simulink model "SimulinkMorphEUS"  (R2025a)
settings: Solver=VariableStepAuto  StartTime=0.0  StopTime=Tfinal  RelTol=1e-3
values from neighbouring files (symbols this model uses):
  Ixx = 0.246    [SetDroneControl(5).m]    (also in SetDroneControl.m)
  Iyy = 0.336    [SetDroneControl(5).m]    (also in SetDroneControl.m)
  Izz = 0.234    [SetDroneControl(5).m]    (also in SetDroneControl.m)
  lx = 0.2125    [SetDroneControl(5).m]    (also in SetDroneControl.m)
  ly = 0.2125    [SetDroneControl(5).m]    (also in SetDroneControl.m)
  Mass = 3    [SetDroneControl(5).m]    (also in SetDroneControl.m = 5)
libraries: slpidlib x12, matrix_library x8, robotcorelib x4, aerolibobsolete x1, uavutilslib x1
(part 1 of 2)
settings Model: Creator=Nguyen_Duc  LastModifiedBy=Nguyen_Duc

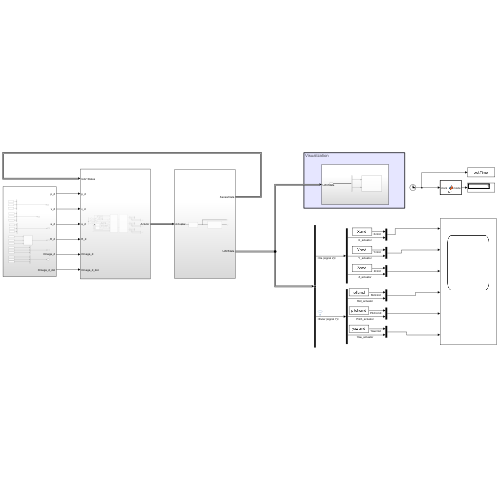
[thumbnail: Simulink's stored preview of the top-level diagram]
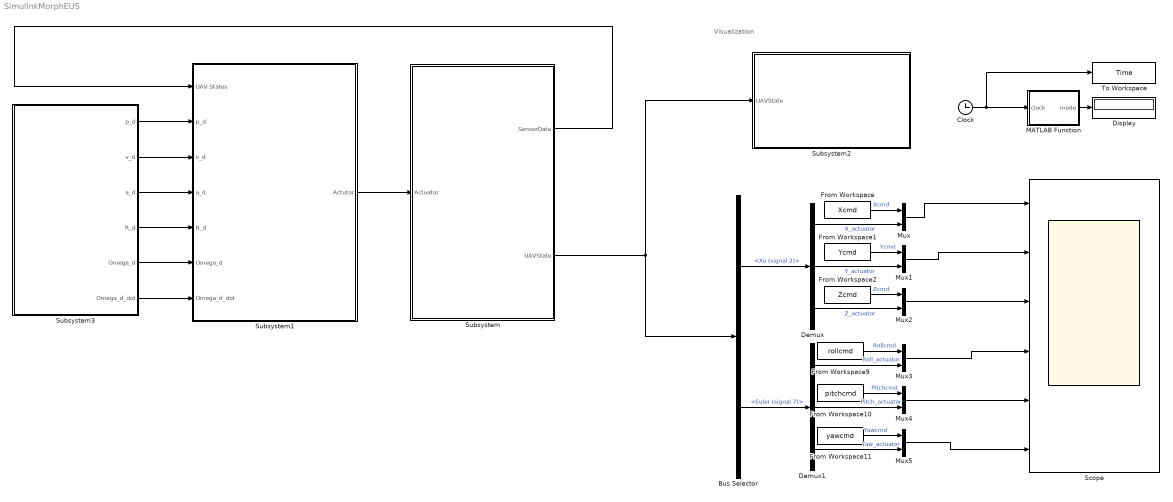
== system SimulinkMorphEUS ==
  note: Visualization
  Bus Selector : BusSelector  OutputSignals=Xe (signal 2),Euler (signal 7)
  Clock : Clock
  Demux : Demux  Outputs=3
  Demux1 : Demux  Outputs=3
  Display : Display
  From Workspace : FromWorkspace  VariableName=Xcmd
  From Workspace1 : FromWorkspace  VariableName=Ycmd
  From Workspace10 : FromWorkspace  VariableName=pitchcmd
  From Workspace11 : FromWorkspace  VariableName=yawcmd
  From Workspace2 : FromWorkspace  VariableName=Zcmd
  From Workspace9 : FromWorkspace  VariableName=rollcmd
  MATLAB Function : MATLAB Function  TreatAsAtomicUnit=on
  Mux{,1..5} (6 alike) : Mux  Inputs=2
  Scope : Scope  NumInputPorts=6
      settings: ActiveDisplayYMinimum=-0.1263691914404973  ActiveDisplayYMaximum=0.14324879526633019
  Subsystem : Subsystem
  Subsystem1 : Subsystem
  Subsystem2 : Subsystem
  Subsystem3 : Subsystem
  To Workspace : ToWorkspace  VariableName=Time  SaveFormat=Timeseries  SampleTime=-1
  wires:
  Subsystem/2(UAVState) -> Subsystem2/1(UAVState), Bus Selector/1
  Subsystem1/1(Actutor) -> Subsystem/1(Actuator)
  Subsystem/1(SensorData) -> Subsystem1/1(UAV States)
  Clock/1 -> To Workspace/1, MATLAB Function/1(clock)
  MATLAB Function/1(mode) -> Display/1
  Subsystem3/1(p_d) -> Subsystem1/2(p_d)
  Subsystem3/2(v_d) -> Subsystem1/3(v_d)
  Subsystem3/3(a_d) -> Subsystem1/4(a_d)
  Subsystem3/4(R_d) -> Subsystem1/5(R_d)
  Subsystem3/5(Omega_d) -> Subsystem1/6(Omega_d)
  Subsystem3/6(Omega_d_dot) -> Subsystem1/7(Omega_d_dot)
  Bus Selector/1 -> Demux/1  "<Xe (signal 2)>"
  Demux/1 -> Mux/2  "X_actuator"
  From Workspace/1 -> Mux/1  "Xcmd"
  Mux/1 -> Scope/1
  Demux/2 -> Mux1/2  "Y_actuator"
  From Workspace1/1 -> Mux1/1  "Ycmd"
  Mux1/1 -> Scope/2
  From Workspace2/1 -> Mux2/1  "Zcmd"
  Demux/3 -> Mux2/2  "Z_actuator"
  Mux2/1 -> Scope/3
  From Workspace11/1 -> Mux5/1  "Yawcmd"
  Mux5/1 -> Scope/6
  Mux3/1 -> Scope/4
  Mux4/1 -> Scope/5
  From Workspace10/1 -> Mux4/1  "Pitchcmd"
  Demux1/3 -> Mux5/2  "Yaw_actuator"
  Demux1/1 -> Mux3/2  "Roll_actuator"
  Demux1/2 -> Mux4/2  "Pitch_actuator"
  From Workspace9/1 -> Mux3/1  "Rollcmd"
  Bus Selector/2 -> Demux1/1  "<Euler (signal 7)>"

== system SimulinkMorphEUS/Subsystem ==
  Actuator : Inport
  MorphEUS Dynamics : Subsystem
  Subsystem : Subsystem
  SensorData : Outport
  UAVState : Outport  Port=2
  wires:
  Actuator/1 -> MorphEUS Dynamics/1(Actuator)
  Subsystem/1(SensorData) -> SensorData/1
  MorphEUS Dynamics/1(States) -> Subsystem/1(UAVStates), UAVState/1  "Ground Truth"

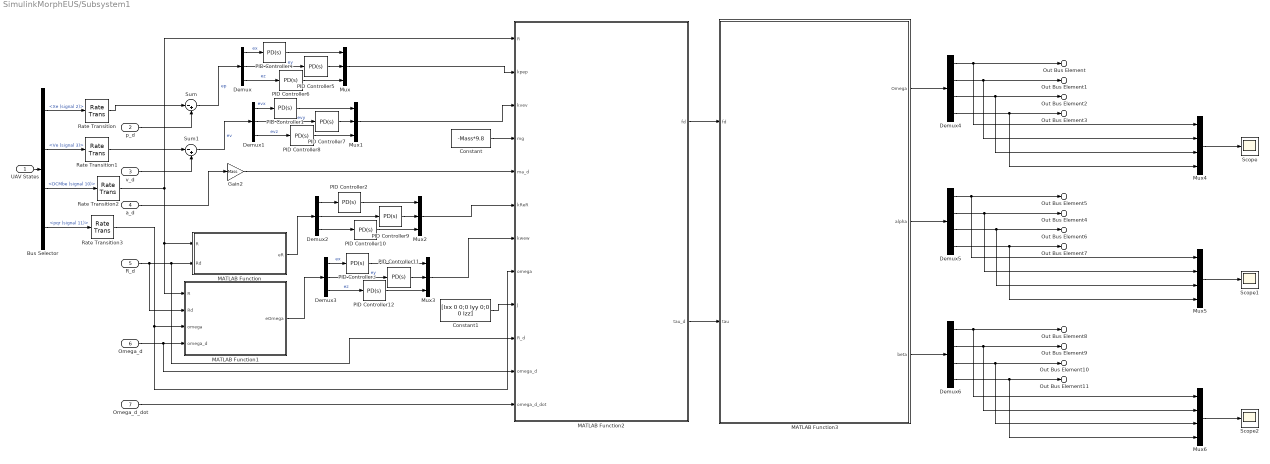
== system SimulinkMorphEUS/Subsystem1 ==
  UAV States : Inport
  p_d : Inport  Port=2
  v_d : Inport  Port=3
  a_d : Inport  Port=4
  R_d : Inport  Port=5
  Omega_d : Inport  Port=6
  Omega_d_dot : Inport  Port=7
  Bus Selector : BusSelector  OutputSignals=Xe (signal 2),Ve (signal 3),DCMbe (signal 10),pqr (signal 11)
  Constant : Constant  Value=-Mass*9.8
  Constant1 : Constant  Value=[Ixx 0 0;0 Iyy 0;0 0 Izz]
  Demux{,1..3} (4 alike) : Demux  Outputs=3
  Demux4 : Demux
  Demux5 : Demux
  Demux6 : Demux
  Gain2 : Gain  Gain=Mass
  MATLAB Function : MATLAB Function  TreatAsAtomicUnit=on
  MATLAB Function1 : MATLAB Function  TreatAsAtomicUnit=on
  MATLAB Function2 : MATLAB Function  TreatAsAtomicUnit=on
  MATLAB Function3 : MATLAB Function  TreatAsAtomicUnit=on
  Mux{,1..3} (4 alike) : Mux  Inputs=3
  Mux4 : Mux
  Mux5 : Mux
  Mux6 : Mux
  PID Controller{1..12} (12 alike) : slpidlib/PID Controller  Controller=PD  Form=Parallel  TimeDomain=Continuous-time  UseExternalTs=off  SampleTime=-1  IntegratorMethod=Forward Euler  FilterMethod=Forward Euler  ControllerParametersSource=internal  P=5  I=1  UseKiTs=off  D=0  UseExternalDerivativeSource=off  N=100  UseFilter=on  TunerSelectOption=Transfer Function Based (PID Tuner App)  InitialConditionSource=internal  InitialConditionForIntegrator=0  InitialConditionForFilter=0  DifferentiatorICPrevScaledInput=0  ExternalReset=none  TrackingMode=off  Kt=1  LimitOutput=off  SatLimitsSource=internal  UpperSaturationLimit=inf  LowerSaturationLimit=-inf  LinearizeAsGain=on  AntiWindupMode=none  Kb=1  LimitIntegrator=off  UpperIntegratorSaturationLimit=inf  LowerIntegratorSaturationLimit=-inf  POutMin=[]  POutMax=[]  IOutMin=[]  IOutMax=[]  DOutMin=[]  DOutMax=[]  NOutMin=[]  NOutMax=[]  SumOutMin=[]  SumOutMax=[]  SaturationOutMin=[]  SaturationOutMax=[]  PParamMin=[]  PParamMax=[]  IParamMin=[]  IParamMax=[]  DParamMin=[]  DParamMax=[]  NParamMin=[]  NParamMax=[]  KbParamMin=[]  KbParamMax=[]  KtParamMin=[]  KtParamMax=[]  KbOutMin=[]  KbOutMax=[]  KtOutMin=[]  KtOutMax=[]  IntegratorOutMin=[]  IntegratorOutMax=[]  FilterOutMin=[]  FilterOutMax=[]  SumI1OutMin=[]  SumI1OutMax=[]  SumI2OutMin=[]  SumI2OutMax=[]  SumI3OutMin=[]  SumI3OutMax=[]  SumI4OutMin=[]  SumI4OutMax=[]  SumDOutMin=[]  SumDOutMax=[]  DifferentiatorOutMin=[]  DifferentiatorOutMax=[]  FilterDiffOutCoefMin=[]  FilterDiffOutCoefMax=[]  ReciprocalOutMin=[]  ReciprocalOutMax=[]  SumDenOutMin=[]  SumDenOutMax=[]  SumNumOutMin=[]  SumNumOutMax=[]  DivideOutMin=[]  DivideOutMax=[]  UdiffTsProdOutMin=[]  UdiffTsProdOutMax=[]  NTsProdOutMin=[]  NTsProdOutMax=[]  UintegralTsProdOutMin=[]  UintegralTsProdOutMax=[]  UngainTsProdOutMin=[]  UngainTsProdOutMax=[]  ClampingZeroOutDataTypeStr=Inherit: Inherit via back propagation  ClampingZeroOutMin=[]  ClampingZeroOutMax=[]  FilterDenConstantOutDataTypeStr=Inherit: Inherit via back propagation  FilterDenConstantOutMin=[]  FilterDenConstantOutMax=[]  PCopyOutDataTypeStr=Inherit: Inherit via back propagation  PCopyOutMin=[]  PCopyOutMax=[]  NCopyOutDataTypeStr=Inherit: Inherit via back propagation  NCopyOutMin=[]  NCopyOutMax=[]  IntegratorContinuousStateAttributes=''  IntegratorStateMustResolveToSignalObject=off  IntegratorRTWStateStorageClass=Auto  FilterContinuousStateAttributes=''  FilterStateMustResolveToSignalObject=off  FilterRTWStateStorageClass=Auto  ParallelPVariant=InternalParameters  IdealPVariant=Disabled  IVariant=Disabled  DVariant=InternalParameters  IntegratorVariant=Disabled  SatVariant=Disabled  AWVariant=Disabled  PCopyVariant=Disabled  TRVariant=Disabled  FdbkBlocksVariant=Forward  IdealPFdbkVariant=Disabled  SatFdbkVariant=Disabled  DerivativeFilterVariant=ContFilter  NVariant=InternalParameters  NCopyVariant=Disabled  FilterICVariant=InternalICsFilter  IntegratorICVariant=Disabled  ExternalResetVariant=Disabled  TRSumVariant=Passthrough  SumFdbkVariant=Disabled  SumVariant=Sum_PD  TsampFilterVariant=InternalTs  TsampNgainVariant=Passthrough  TsampIntegralVariant=Disabled_SignalSpec  ExternalSaturationOutDataTypeStr=Inherit: Same as second input  DerivativeSourceVariant=ErrorSignal  PreIntVariant=InternalPreInt
  Rate Transition{,1..3} (4 alike) : RateTransition  OutPortSampleTime=tss
  Scope : Scope
      settings: ActiveDisplayYMinimum=15.734092150447644  ActiveDisplayYMaximum=26.649109320709051  DataLoggingVariableName=ScopeData2
  Scope1 : Scope
      settings: ActiveDisplayYMinimum=-7.46045590481177  ActiveDisplayYMaximum=5.3328354419928372  DataLoggingVariableName=ScopeData3
  Scope2 : Scope
      settings: ActiveDisplayYMinimum=-1.2276221788236448  ActiveDisplayYMaximum=0.57847317932008258  DataLoggingVariableName=ScopeData4
  Sum : Sum  Inputs=|-+
  Sum1 : Sum  Inputs=|-+
  Out Bus Element : Outport  PortName=Actutor  Element=w1
  Out Bus Element1 : Outport  PortName=Actutor  Element=w2
  Out Bus Element2 : Outport  PortName=Actutor  Element=w3
  Out Bus Element3 : Outport  PortName=Actutor  Element=w4
  Out Bus Element5 : Outport  PortName=Actutor  Element=Alpha1
  Out Bus Element4 : Outport  PortName=Actutor  Element=Alpha2
  Out Bus Element6 : Outport  PortName=Actutor  Element=Alpha3
  Out Bus Element7 : Outport  PortName=Actutor  Element=Alpha4
  Out Bus Element8 : Outport  PortName=Actutor  Element=Beta1
  Out Bus Element9 : Outport  PortName=Actutor  Element=Beta2
  Out Bus Element10 : Outport  PortName=Actutor  Element=Beta3
  Out Bus Element11 : Outport  PortName=Actutor  Element=Beta4
  wires:
  p_d/1 -> Sum/2
  Bus Selector/2 -> Rate Transition1/1  "<Ve (signal 3)>"
  v_d/1 -> Sum1/2
  Sum/1 -> Demux/1  "ep"
  Sum1/1 -> Demux1/1  "ev"
  Bus Selector/3 -> Rate Transition2/1  "<DCMbe (signal 10)>"
  R_d/1 -> MATLAB Function1/2(Rd), MATLAB Function2/10(R_d), MATLAB Function/2(Rd)
  Omega_d/1 -> MATLAB Function2/11(omega_d), MATLAB Function1/4(omega_d)
  MATLAB Function/1(eR) -> Demux2/1
  MATLAB Function1/1(eOmega) -> Demux3/1
  Mux/1 -> MATLAB Function2/2(kpep)
  Constant/1 -> MATLAB Function2/4(mg)
  a_d/1 -> Gain2/1
  Gain2/1 -> MATLAB Function2/5(ma_d)
  Omega_d_dot/1 -> MATLAB Function2/12(omega_d_dot)
  Constant1/1 -> MATLAB Function2/9(J)
  Demux/1 -> PID Controller4/1  "ex"
  Demux/3 -> PID Controller6/1  "ez"
  Demux/2 -> PID Controller5/1  "ey"
  PID Controller5/1 -> Mux/2
  PID Controller6/1 -> Mux/3
  PID Controller4/1 -> Mux/1
  Demux1/3 -> PID Controller8/1  "evz"
  Demux1/2 -> PID Controller7/1  "evy"
  PID Controller1/1 -> Mux1/1
  PID Controller8/1 -> Mux1/3
  Demux1/1 -> PID Controller1/1  "evx"
  PID Controller7/1 -> Mux1/2
  Mux1/1 -> MATLAB Function2/3(kvev)
  Demux2/3 -> PID Controller10/1
  Demux2/2 -> PID Controller9/1
  PID Controller2/1 -> Mux2/1
  PID Controller10/1 -> Mux2/3
  Demux2/1 -> PID Controller2/1
  PID Controller9/1 -> Mux2/2
  Mux2/1 -> MATLAB Function2/6(kReR)
  Demux3/3 -> PID Controller12/1  "ez"
  Demux3/2 -> PID Controller11/1  "ey"
  PID Controller3/1 -> Mux3/1
  PID Controller12/1 -> Mux3/3
  Demux3/1 -> PID Controller3/1  "ex"
  PID Controller11/1 -> Mux3/2
  Mux3/1 -> MATLAB Function2/7(kwew)
  MATLAB Function2/1(fd) -> MATLAB Function3/1(fd)
  MATLAB Function2/2(tau_d) -> MATLAB Function3/2(tau)
  MATLAB Function3/1(Omega) -> Demux4/1
  Demux4/1 -> Mux4/1, Out Bus Element/1
  Demux4/2 -> Mux4/2, Out Bus Element1/1
  Demux4/3 -> Mux4/3, Out Bus Element2/1
  Demux4/4 -> Mux4/4, Out Bus Element3/1
  MATLAB Function3/2(alpha) -> Demux5/1
  MATLAB Function3/3(beta) -> Demux6/1
  UAV States/1 -> Bus Selector/1
  Bus Selector/4 -> Rate Transition3/1  "<pqr (signal 11)>"
  Bus Selector/1 -> Rate Transition/1  "<Xe (signal 2)>"
  Mux4/1 -> Scope/1
  Mux5/1 -> Scope1/1
  Demux5/2 -> Mux5/2, Out Bus Element4/1
  Demux5/3 -> Mux5/3, Out Bus Element6/1
  Demux5/1 -> Mux5/1, Out Bus Element5/1
  Demux5/4 -> Mux5/4, Out Bus Element7/1
  Mux6/1 -> Scope2/1
  Demux6/2 -> Mux6/2, Out Bus Element9/1
  Demux6/3 -> Mux6/3, Out Bus Element10/1
  Demux6/1 -> Mux6/1, Out Bus Element8/1
  Demux6/4 -> Mux6/4, Out Bus Element11/1
  Rate Transition/1 -> Sum/1
  Rate Transition1/1 -> Sum1/1
  Rate Transition2/1 -> MATLAB Function2/1(R), MATLAB Function/1(R), MATLAB Function1/1(R)
  Rate Transition3/1 -> MATLAB Function2/8(omega), MATLAB Function1/3(omega)

== system SimulinkMorphEUS/Subsystem2 ==
  UAVState : Inport
  Bus Selector : BusSelector  OutputSignals=Xe (signal 2),pqr (signal 11)
  Trajectory : uavutilslib/UAV Animation  NumUAV=1  DynamicUAVConfig=off  UAVType=Multirotor  UAVSize=5  UAVColor=[1 0 0]  UAVTrajectoryAlpha=1  InertialZDirection=Down  RotationFormat=Euler ZYX  DrawMarkers=off  SampleTime=0.1
  wires:
  UAVState/1 -> Bus Selector/1
  Bus Selector/1 -> Trajectory/1  "<Xe (signal 2)>"
  Bus Selector/2 -> Trajectory/2  "<pqr (signal 11)>"

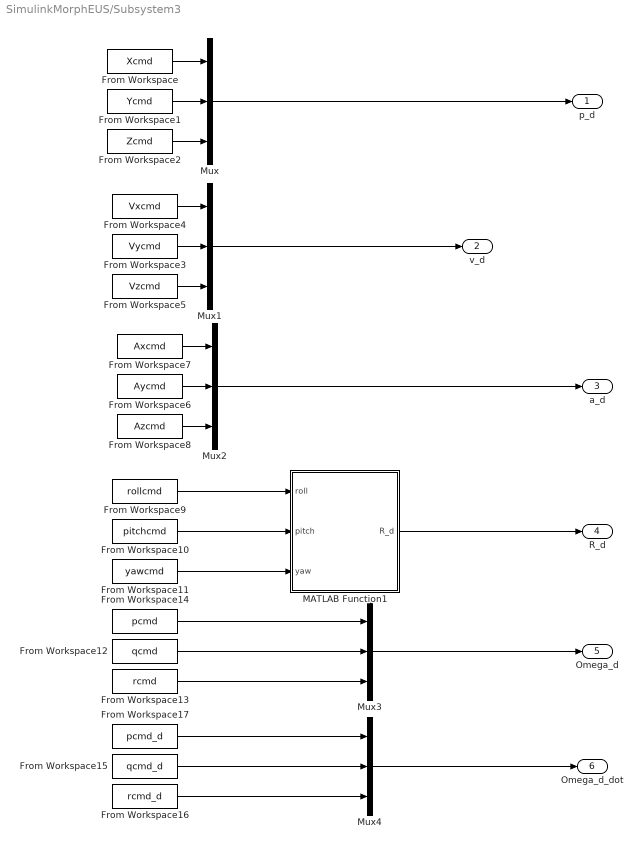
== system SimulinkMorphEUS/Subsystem3 ==
  From Workspace : FromWorkspace  VariableName=Xcmd
  From Workspace1 : FromWorkspace  VariableName=Ycmd
  From Workspace10 : FromWorkspace  VariableName=pitchcmd
  From Workspace11 : FromWorkspace  VariableName=yawcmd
  From Workspace12 : FromWorkspace  VariableName=qcmd
  From Workspace13 : FromWorkspace  VariableName=rcmd
  From Workspace14 : FromWorkspace  VariableName=pcmd
  From Workspace15 : FromWorkspace  VariableName=qcmd_d
  From Workspace16 : FromWorkspace  VariableName=rcmd_d
  From Workspace17 : FromWorkspace  VariableName=pcmd_d
  From Workspace2 : FromWorkspace  VariableName=Zcmd
  From Workspace3 : FromWorkspace  VariableName=Vycmd
  From Workspace4 : FromWorkspace  VariableName=Vxcmd
  From Workspace5 : FromWorkspace  VariableName=Vzcmd
  From Workspace6 : FromWorkspace  VariableName=Aycmd
  From Workspace7 : FromWorkspace  VariableName=Axcmd
  From Workspace8 : FromWorkspace  VariableName=Azcmd
  From Workspace9 : FromWorkspace  VariableName=rollcmd
  MATLAB Function1 : MATLAB Function  TreatAsAtomicUnit=on
  Mux{,1..4} (5 alike) : Mux  Inputs=3
  p_d : Outport
  v_d : Outport  Port=2
  a_d : Outport  Port=3
  R_d : Outport  Port=4
  Omega_d : Outport  Port=5
  Omega_d_dot : Outport  Port=6
  wires:
  From Workspace/1 -> Mux/1
  From Workspace6/1 -> Mux2/2
  From Workspace1/1 -> Mux/2
  From Workspace11/1 -> MATLAB Function1/3(yaw)
  From Workspace4/1 -> Mux1/1
  Mux/1 -> p_d/1
  From Workspace2/1 -> Mux/3
  From Workspace8/1 -> Mux2/3
  From Workspace7/1 -> Mux2/1
  From Workspace5/1 -> Mux1/3
  From Workspace3/1 -> Mux1/2
  Mux4/1 -> Omega_d_dot/1
  From Workspace15/1 -> Mux4/2
  From Workspace16/1 -> Mux4/3
  Mux3/1 -> Omega_d/1
  From Workspace17/1 -> Mux4/1
  From Workspace13/1 -> Mux3/3
  Mux1/1 -> v_d/1
  From Workspace10/1 -> MATLAB Function1/2(pitch)
  From Workspace14/1 -> Mux3/1
  From Workspace9/1 -> MATLAB Function1/1(roll)
  From Workspace12/1 -> Mux3/2
  MATLAB Function1/1(R_d) -> R_d/1
  Mux2/1 -> a_d/1

== system SimulinkMorphEUS/Subsystem/MorphEUS Dynamics ==
  note: Forces and Moments - VTOL UAV plant model and weather model
      | 6DOF (Euler Angles) - Integrate the six-degrees-of-freedom equations of motion in body axis.
      | Ground Truth Bus - converts UAV States into bus
  Actuator : Inport
  6DOF (Euler Angles) : aerolibobsolete/6DOF (Euler Angles)  units=Metric (MKS)  mtype=Fixed  rep=Euler Angles  xme_0=[0, 0 , 0]  Vm_0=[0, 0 , 0]  eul_0=[0, 0 , 0]  pm_0=[0 0 0]  mass_0=Mass  mass_e=0.5  mass_f=2.0  inertia=[Ixx 0 0; 0 Iyy 0; 0 0 Izz]  inertia_e=eye(3)  inertia_f=2*eye(3)  k_quat=1.0  vre_flag=on  abi_flag=on  aMode=0  xme_statename=''  Vm_statename=''  eul_statename=''  quat_statename=''  pm_statename=''  mass_statename=''
  Feedback : Subsystem
  Ground Truth Bus : Subsystem
  Rate Transition : RateTransition  OutPortSampleTime=tss
  Subsystem : Subsystem
  Terminator : Terminator
  States : Outport
  wires:
  Actuator/1 -> Subsystem/1(Actuator)
  6DOF (Euler Angles)/4 -> Feedback/4(DCMbe), Ground Truth Bus/4(DCMbe)  "DCMbe"
  Subsystem/3(RotorParams) -> Rate Transition/1  "RotorParams"
  Rate Transition/1 -> Ground Truth Bus/9(RotorParams), Feedback/7(RotorParameters)
  6DOF (Euler Angles)/1 -> Feedback/1(Ve), Ground Truth Bus/1(Ve)  "Ve"
  Feedback/1(GroundTruth) -> Subsystem/2(States)
  Subsystem/2(M) -> 6DOF (Euler Angles)/2
  Subsystem/1(F) -> 6DOF (Euler Angles)/1
  6DOF (Euler Angles)/3 -> Feedback/3(Euler), Ground Truth Bus/3(Euler)  "Euler"
  Ground Truth Bus/1(UAV States) -> States/1
  6DOF (Euler Angles)/6 -> Feedback/6(pqr), Ground Truth Bus/6(pqr)  "pqr"
  6DOF (Euler Angles)/5 -> Feedback/5(Vb), Ground Truth Bus/5(Vb)  "Vb"
  6DOF (Euler Angles)/2 -> Feedback/2(Xe), Ground Truth Bus/2(Xe)  "Xe"
  6DOF (Euler Angles)/7 -> Terminator/1
  6DOF (Euler Angles)/9 -> Ground Truth Bus/8(Abe)
  6DOF (Euler Angles)/8 -> Ground Truth Bus/7(Abb)

== system SimulinkMorphEUS/Subsystem/Subsystem ==
  UAVStates : Inport
  Rate Transition : RateTransition  OutPortSampleTime=0.005
  SensorData : Outport
  wires:
  UAVStates/1 -> Rate Transition/1
  Rate Transition/1 -> SensorData/1

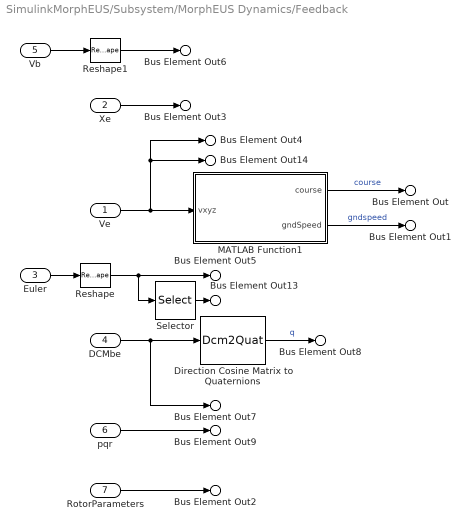
== system SimulinkMorphEUS/Subsystem/MorphEUS Dynamics/Feedback ==
  Ve : Inport
  Xe : Inport  Port=2
  Euler : Inport  Port=3
  DCMbe : Inport  Port=4
  Vb : Inport  Port=5
  pqr : Inport  Port=6
  RotorParameters : Inport  Port=7
  Direction Cosine Matrix to Quaternions : Dcm2Quat
  MATLAB Function1 : MATLAB Function  TreatAsAtomicUnit=on
  Reshape : Reshape  OutputDimensionality=Column vector (2-D)
  Reshape1 : Reshape  OutputDimensionality=Row vector (2-D)
  Selector : Selector  InputPortWidth=3  IndexOptions=Index vector (dialog)  Indices=[3 2 1]  OutputSizes=1
  Bus Element Out : Outport  PortName=GroundTruth  Element=course
  Bus Element Out1 : Outport  PortName=GroundTruth  Element=gndspeed
  Bus Element Out3 : Outport  PortName=GroundTruth  Element=Xe
  Bus Element Out4 : Outport  PortName=GroundTruth  Element=Ve
  Bus Element Out7 : Outport  PortName=GroundTruth  Element=DCMbe
  Bus Element Out8 : Outport  PortName=GroundTruth  Element=q
  Bus Element Out9 : Outport  PortName=GroundTruth  Element=pqr
  Bus Element Out6 : Outport  PortName=GroundTruth  Element=Vb
  Bus Element Out5 : Outport  PortName=GroundTruth  Element=Euler
  Bus Element Out13 : Outport  PortName=GroundTruth  Element=ypr
  Bus Element Out14 : Outport  PortName=GroundTruth  Element=Ve_ground
  Bus Element Out2 : Outport  PortName=GroundTruth  Element=RotorParameters
  wires:
  Reshape1/1 -> Bus Element Out6/1
  Reshape/1 -> Bus Element Out5/1, Selector/1
  Selector/1 -> Bus Element Out13/1
  pqr/1 -> Bus Element Out9/1
  Direction Cosine Matrix to Quaternions/1 -> Bus Element Out8/1  "q"
  Vb/1 -> Reshape1/1
  Euler/1 -> Reshape/1
  Xe/1 -> Bus Element Out3/1
  MATLAB Function1/2(gndSpeed) -> Bus Element Out1/1  "gndspeed"
  MATLAB Function1/1(course) -> Bus Element Out/1  "course"
  Ve/1 -> MATLAB Function1/1(vxyz), Bus Element Out4/1, Bus Element Out14/1
  DCMbe/1 -> Direction Cosine Matrix to Quaternions/1, Bus Element Out7/1
  RotorParameters/1 -> Bus Element Out2/1

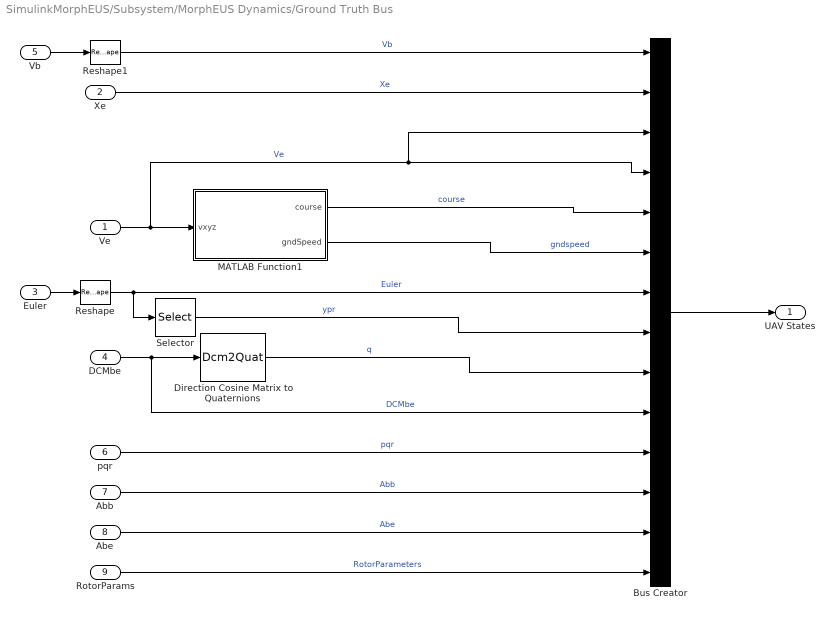
== system SimulinkMorphEUS/Subsystem/MorphEUS Dynamics/Ground Truth Bus ==
  Ve : Inport
  Xe : Inport  Port=2
  Euler : Inport  Port=3
  DCMbe : Inport  Port=4
  Vb : Inport  Port=5
  pqr : Inport  Port=6
  Abb : Inport  Port=7
  Abe : Inport  Port=8
  RotorParams : Inport  Port=9
  Bus Creator : BusCreator  Inputs=14
  Direction Cosine Matrix to Quaternions : Dcm2Quat
  MATLAB Function1 : MATLAB Function  TreatAsAtomicUnit=on
  Reshape : Reshape  OutputDimensionality=Column vector (2-D)
  Reshape1 : Reshape  OutputDimensionality=Row vector (2-D)
  Selector : Selector  InputPortWidth=3  IndexOptions=Index vector (dialog)  Indices=[3 2 1]  OutputSizes=1
  UAV States : Outport
  wires:
  DCMbe/1 -> Bus Creator/10, Direction Cosine Matrix to Quaternions/1  "DCMbe"
  Ve/1 -> Bus Creator/4, Bus Creator/3, MATLAB Function1/1(vxyz)  "Ve"
  MATLAB Function1/1(course) -> Bus Creator/5  "course"
  MATLAB Function1/2(gndSpeed) -> Bus Creator/6  "gndspeed"
  Xe/1 -> Bus Creator/2  "Xe"
  Euler/1 -> Reshape/1
  Vb/1 -> Reshape1/1
  Direction Cosine Matrix to Quaternions/1 -> Bus Creator/9  "q"
  pqr/1 -> Bus Creator/11  "pqr"
  Abb/1 -> Bus Creator/12  "Abb"
  Abe/1 -> Bus Creator/13  "Abe"
  RotorParams/1 -> Bus Creator/14  "RotorParameters"
  Selector/1 -> Bus Creator/8  "ypr"
  Reshape/1 -> Bus Creator/7, Selector/1  "Euler"
  Reshape1/1 -> Bus Creator/1  "Vb"
  Bus Creator/1 -> UAV States/1

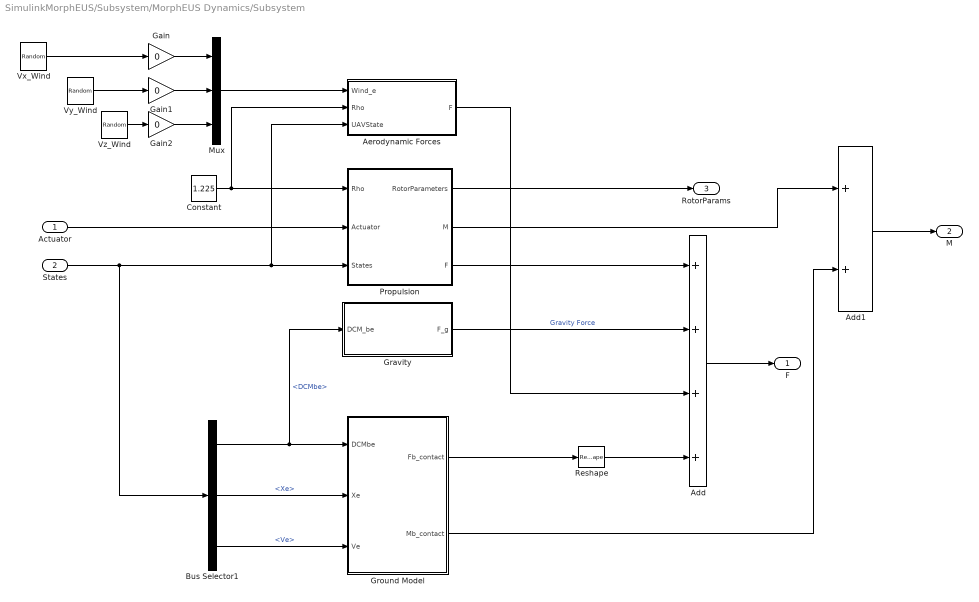
== system SimulinkMorphEUS/Subsystem/MorphEUS Dynamics/Subsystem ==
  Actuator : Inport
  States : Inport  Port=2
  Add : Sum  Inputs=++++
  Add1 : Sum
  Aerodynamic Forces : Subsystem
  Bus Selector1 : BusSelector  OutputSignals=DCMbe,Xe,Ve
  Constant : Constant  Value=1.225
  Gain : Gain  Gain=0
  Gain1 : Gain  Gain=0
  Gain2 : Gain  Gain=0
  Gravity : Subsystem
  Ground Model : Subsystem  VariantControl=Groundon==1
  Mux : Mux  Inputs=3
  Propulsion : Subsystem
  Reshape : Reshape
  Vx_Wind : UniformRandomNumber  SampleTime=0.1
  Vy_Wind : UniformRandomNumber  SampleTime=0.1
  Vz_Wind : UniformRandomNumber  SampleTime=0.1
  F : Outport
  M : Outport  Port=2
  RotorParams : Outport  Port=3
  wires:
  Vx_Wind/1 -> Gain/1
  Constant/1 -> Aerodynamic Forces/2(Rho), Propulsion/1(Rho)
  Gain2/1 -> Mux/3
  States/1 -> Bus Selector1/1, Aerodynamic Forces/3(UAVState), Propulsion/3(States)
  Ground Model/2(Mb_contact) -> Add1/2
  Propulsion/1(RotorParameters) -> RotorParams/1
  Propulsion/3(F) -> Add/1
  Gain1/1 -> Mux/2
  Aerodynamic Forces/1(F) -> Add/3
  Bus Selector1/2 -> Ground Model/2(Xe)  "<Xe>"
  Bus Selector1/1 -> Gravity/1(DCM_be), Ground Model/1(DCMbe)  "<DCMbe>"
  Add1/1 -> M/1
  Actuator/1 -> Propulsion/2(Actuator)
  Mux/1 -> Aerodynamic Forces/1(Wind_e)
  Vz_Wind/1 -> Gain2/1
  Vy_Wind/1 -> Gain1/1
  Propulsion/2(M) -> Add1/1
  Gravity/1(F_g) -> Add/2  "Gravity Force"
  Add/1 -> F/1
  Ground Model/1(Fb_contact) -> Reshape/1
  Bus Selector1/3 -> Ground Model/3(Ve)  "<Ve>"
  Reshape/1 -> Add/4
  Gain/1 -> Mux/1

== system SimulinkMorphEUS/Subsystem/MorphEUS Dynamics/Subsystem/Aerodynamic Forces ==
  note: The drag equation quantifies the drag force on a UAV:
      | F = 0.5 * ρ * V² * Cd * A : F : Drag force
      | ρ (rho) : Air density
      | V : Velocity of the UAV
      | Cd : Drag coefficient
      | A : Reference area
  Wind_e : Inport
  Rho : Inport  Port=2
  UAVState : Inport  Port=3
  Bus Selector2 : BusSelector  OutputSignals=DCMbe,Ve
  Compute Air Data : Subsystem  TreatAsAtomicUnit=on  VariantControl=use_aerospace_blocks == 1
  Matrix Multiply : Product  Multiplication=Matrix(*)
  Vair : Sum  Inputs=+-  InputSameDT=on  SaturateOnIntegerOverflow=on  OutDataTypeStr=Inherit: Same as first input
  F : Outport
  wires:
  Bus Selector2/2 -> Vair/1  "<Ve>"
  UAVState/1 -> Bus Selector2/1
  Compute Air Data/1(F) -> F/1
  Matrix Multiply/1 -> Compute Air Data/1(Vb)
  Rho/1 -> Compute Air Data/2(Rho)
  Vair/1 -> Matrix Multiply/2
  Bus Selector2/1 -> Matrix Multiply/1  "<DCMbe>"
  Wind_e/1 -> Vair/2

== system SimulinkMorphEUS/Subsystem/MorphEUS Dynamics/Subsystem/Gravity ==
  DCM_be : Inport
  Constant : Constant  Value=[0 0 9.806]'
  Gain : Gain  Gain=Mass
  Matrix Multiply : Product  Multiplication=Matrix(*)
  F_g : Outport
  wires:
  Matrix Multiply/1 -> Gain/1
  Constant/1 -> Matrix Multiply/2
  DCM_be/1 -> Matrix Multiply/1
  Gain/1 -> F_g/1

== system SimulinkMorphEUS/Subsystem/MorphEUS Dynamics/Subsystem/Ground Model ==
  note: Body is assumed to be a rigid point mass on ground for contact force calculations.
      |
      | Normal force is modelled as a spring mass damper.
      |
      | Friction is modelled using Soft Coulomb model.
  DCMbe : Inport
  Xe : Inport  Port=2
  Ve : Inport  Port=3
  Constant : Constant  Value=[0 0 0]  SampleTime=-1
  Friction Force : Subsystem
  Matrix Multiply : Product  Multiplication=Matrix(*)
  Mux1 : Mux  Inputs=2
  Normal Force : Subsystem
  Selector : Selector  InputPortWidth=3  IndexOptions=Index vector (dialog)  Indices=[3]  OutputSizes=1
  Selector1 : Selector  InputPortWidth=3  IndexOptions=Index vector (dialog)  Indices=[3]  OutputSizes=1
  Selector2 : Selector  InputPortWidth=3  IndexOptions=Index vector (dialog)  Indices=[1,2]  OutputSizes=1
  Unary Minus1 : UnaryMinus
  Fb_contact : Outport
  Mb_contact : Outport  Port=2
  wires:
  Xe/1 -> Selector/1
  Ve/1 -> Selector2/1, Selector1/1
  Selector1/1 -> Normal Force/1(Vz)
  Selector/1 -> Normal Force/2(Z)
  DCMbe/1 -> Matrix Multiply/1
  Matrix Multiply/1 -> Fb_contact/1
  Normal Force/1(Normal) -> Friction Force/2(Fn), Unary Minus1/1
  Mux1/1 -> Matrix Multiply/2
  Unary Minus1/1 -> Mux1/2
  Selector2/1 -> Friction Force/1(V)
  Friction Force/1(Friction) -> Mux1/1
  Constant/1 -> Mb_contact/1

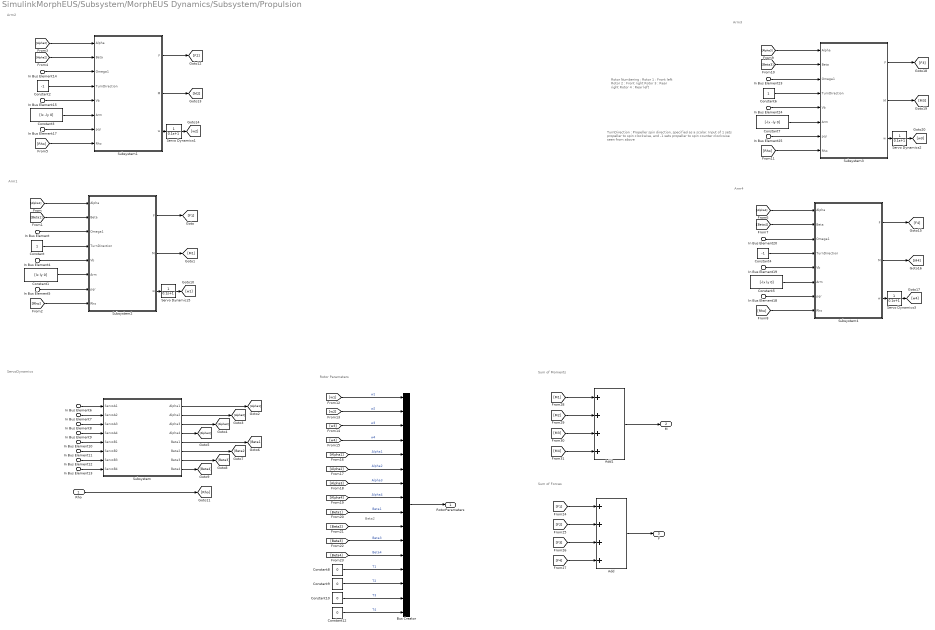
== system SimulinkMorphEUS/Subsystem/MorphEUS Dynamics/Subsystem/Propulsion ==
  note: Beta2
  note: Arm2
  note: ServoDynamics
  note: Rotor Numbering :
      | Rotor 1 : Front left
      | Rotor 2 : Front right
      | Rotor 3 : Rear right
      | Rotor 4 : Rear left
  note: TurnDirection : Propeller spin direction, specified as a scalar. Input of 1 sets propeller to spin clockwise, and -1 sets propeller to spin counter clockwise seen from above
  note: Arm1
  note: Arm3
  note: Arm4
  note: Rotor Parameters
  note: Sum of Moments
  note: Sum of Forces
  Rho : Inport
  In Bus Element : Inport  Port=2  PortName=Actuator  Element=w1
  In Bus Element14 : Inport  Port=2  PortName=Actuator  Element=w2
  In Bus Element23 : Inport  Port=2  PortName=Actuator  Element=w3
  In Bus Element20 : Inport  Port=2  PortName=Actuator  Element=w4
  In Bus Element6 : Inport  Port=2  PortName=Actuator  Element=Alpha1
  In Bus Element7 : Inport  Port=2  PortName=Actuator  Element=Alpha2
  In Bus Element8 : Inport  Port=2  PortName=Actuator  Element=Alpha3
  In Bus Element9 : Inport  Port=2  PortName=Actuator  Element=Alpha4
  In Bus Element10 : Inport  Port=2  PortName=Actuator  Element=Beta1
  In Bus Element11 : Inport  Port=2  PortName=Actuator  Element=Beta2
  In Bus Element12 : Inport  Port=2  PortName=Actuator  Element=Beta3
  In Bus Element13 : Inport  Port=2  PortName=Actuator  Element=Beta4
  In Bus Element{4,15,19,24} (4 alike) : Inport  Port=3  PortName=States  Element=Vb
  In Bus Element{5,17..18,25} (4 alike) : Inport  Port=3  PortName=States  Element=pqr
  Add : Sum  Inputs=++++
  Add1 : Sum  Inputs=++++
  Bus Creator : BusCreator  Inputs=16
  Constant : Constant
  Constant1 : Constant  Value=[lx ly 0]
  Constant{8..10,12} (4 alike) : Constant  Value=0
  Constant2 : Constant  Value=-1
  Constant3 : Constant  Value=[lx -ly 0]
  Constant4 : Constant  Value=-1
  Constant5 : Constant  Value=[-lx ly 0]
  Constant6 : Constant
  Constant7 : Constant  Value=[-lx -ly 0]
  Servo Dynamics{1..3,5} (4 alike) : TransferFcn  Denominator=[0.1 1]
  Subsystem : Subsystem
  Subsystem1 : Subsystem
  Subsystem2 : Subsystem
  Subsystem3 : Subsystem
  Subsystem4 : Subsystem
  RotorParameters : Outport
  M : Outport  Port=2
  F : Outport  Port=3
  wires:
  Constant/1 -> Subsystem2/4(TurnDirection)
  Subsystem2/2(M) -> [M1]
  Subsystem2/1(F) -> [F1]
  Constant1/1 -> Subsystem2/6(Arm)
  In Bus Element5/1 -> Subsystem2/7(pqr)
  In Bus Element4/1 -> Subsystem2/5(Vb)
  [Alpha1] -> Subsystem2/1(Alpha)
  [Beta1] -> Subsystem2/2("Beta ")
  In Bus Element/1 -> Subsystem2/3(Omega1)
  In Bus Element6/1 -> Subsystem/1(ServoA1)
  In Bus Element7/1 -> Subsystem/2(ServoA2)
  In Bus Element8/1 -> Subsystem/3(ServoA3)
  In Bus Element9/1 -> Subsystem/4(ServoA4)
  In Bus Element10/1 -> Subsystem/5(ServoB1)
  In Bus Element11/1 -> Subsystem/6(ServoB2)
  In Bus Element12/1 -> Subsystem/7(ServoB3)
  In Bus Element13/1 -> Subsystem/8(ServoB4)
  Subsystem/1(Alpha1) -> [Alpha1]
  Subsystem/2(Alpha2) -> [Alpha2]
  Subsystem/3(Alpha3) -> [Alpha3]
  Subsystem/4(Alpha4) -> [Alpha4]
  Subsystem/5(Beta1) -> [Beta1]
  Subsystem/7(Beta3) -> [Beta3]
  Subsystem/6(Beta2) -> [Beta2]
  Subsystem/8(Beta4) -> [Beta4]
  Subsystem2/3(w) -> Servo Dynamics5/1
  Servo Dynamics5/1 -> [w1]
  Rho/1 -> [Rho]
  [Rho] -> Subsystem2/8(Rho)
  In Bus Element17/1 -> Subsystem1/7(pqr)
  Subsystem1/3(w) -> Servo Dynamics1/1
  [Rho] -> Subsystem1/8(Rho)
  Servo Dynamics1/1 -> [w2]
  [Alpha2] -> Subsystem1/1(Alpha)
  Constant3/1 -> Subsystem1/6(Arm)
  Subsystem1/1(F) -> [F2]
  Constant2/1 -> Subsystem1/4(TurnDirection)
  In Bus Element15/1 -> Subsystem1/5(Vb)
  Subsystem1/2(M) -> [M2]
  [Alpha2] -> Subsystem1/2("Beta ")
  In Bus Element14/1 -> Subsystem1/3(Omega1)
  In Bus Element18/1 -> Subsystem4/7(pqr)
  Subsystem4/3(w) -> Servo Dynamics3/1
  In Bus Element24/1 -> Subsystem3/5(Vb)
  [Rho] -> Subsystem4/8(Rho)
  Servo Dynamics3/1 -> [w4]
  In Bus Element19/1 -> Subsystem4/5(Vb)
  Constant6/1 -> Subsystem3/4(TurnDirection)
  Subsystem3/1(F) -> [F3]
  Constant7/1 -> Subsystem3/6(Arm)
  Servo Dynamics2/1 -> [w3]
  [Beta3] -> Subsystem3/2("Beta ")
  [Rho] -> Subsystem3/8(Rho)
  Subsystem3/3(w) -> Servo Dynamics2/1
  In Bus Element25/1 -> Subsystem3/7(pqr)
  [Alpha4] -> Subsystem4/1(Alpha)
  Constant5/1 -> Subsystem4/6(Arm)
  Subsystem4/1(F) -> [F4]
  Constant4/1 -> Subsystem4/4(TurnDirection)
  In Bus Element23/1 -> Subsystem3/3(Omega1)
  Subsystem4/2(M) -> [M4]
  Subsystem3/2(M) -> [M3]
  [Beta4] -> Subsystem4/2("Beta ")
  In Bus Element20/1 -> Subsystem4/3(Omega1)
  [Alpha3] -> Subsystem3/1(Alpha)
  [w2] -> Bus Creator/2  "w2"
  [Alpha2] -> Bus Creator/6  "Alpha2"
  Constant10/1 -> Bus Creator/15  "T3"
  [Alpha1] -> Bus Creator/5  "Alpha1"
  [w4] -> Bus Creator/4  "w4"
  Constant12/1 -> Bus Creator/16  "T4"
  Constant8/1 -> Bus Creator/13  "T1"
  Bus Creator/1 -> RotorParameters/1
  [w1] -> Bus Creator/1  "w1"
  [w3] -> Bus Creator/3  "w3"
  Constant9/1 -> Bus Creator/14  "T2"
  [Alpha3] -> Bus Creator/7  "Alpha3"
  [Alpha4] -> Bus Creator/8  "Alpha4"
  [Beta3] -> Bus Creator/11  "Beta3"
  [Beta4] -> Bus Creator/12  "Beta4"
  [Beta1] -> Bus Creator/9  "Beta1"
  [Beta2] -> Bus Creator/10
  [M4] -> Add1/4
  Add1/1 -> M/1
  [F4] -> Add/4
  [F1] -> Add/1
  [F2] -> Add/2
  Add/1 -> F/1
  [M2] -> Add1/2
  [M1] -> Add1/1
  [F3] -> Add/3
  [M3] -> Add1/3

== system SimulinkMorphEUS/Subsystem/MorphEUS Dynamics/Subsystem/Aerodynamic Forces/Compute Air Data ==
  Vb : Inport  PortDimensions=3
  Rho : Inport  Port=2
  MATLAB Function : MATLAB Function  TreatAsAtomicUnit=on
  Terminator : Terminator
  F : Outport
  wires:
  Vb/1 -> MATLAB Function/1(v)
  Rho/1 -> Terminator/1
  MATLAB Function/1(F) -> F/1

== system SimulinkMorphEUS/Subsystem/MorphEUS Dynamics/Subsystem/Ground Model/Friction Force ==
  V : Inport
  Fn : Inport  Port=2
  Product : Product
  Soft Coulomb Friction : Subsystem
  Unary Minus : UnaryMinus
  Friction : Outport
  wires:
  Unary Minus/1 -> Friction/1
  Fn/1 -> Product/2
  Soft Coulomb Friction/1(Out1) -> Product/1
  Product/1 -> Unary Minus/1
  V/1 -> Soft Coulomb Friction/1(V)

== system SimulinkMorphEUS/Subsystem/MorphEUS Dynamics/Subsystem/Ground Model/Normal Force ==
  Vz : Inport
  Z : Inport  Port=2
  Add : Sum
  Constant : Constant  Value=0  SampleTime=-1
  Damper : Gain  Gain=-sqrt((1.2893e+05)*Mass)
  Saturation : Saturate  UpperLimit=inf  LowerLimit=0  ZeroCross=off
  Spring Kp : Gain  Gain=-1.2893e+05
  Switch : Switch  Criteria=u2 > Threshold  SaturateOnIntegerOverflow=off  InputSameDT=off
  Unary Minus : UnaryMinus
  Unary Minus1 : UnaryMinus
  Normal : Outport
  wires:
  Add/1 -> Switch/3
  Constant/1 -> Switch/1
  Z/1 -> Unary Minus/1
  Switch/1 -> Saturation/1
  Damper/1 -> Add/2
  Spring Kp/1 -> Add/1
  Vz/1 -> Unary Minus1/1
  Saturation/1 -> Normal/1
  Unary Minus/1 -> Spring Kp/1, Switch/2
  Unary Minus1/1 -> Damper/1

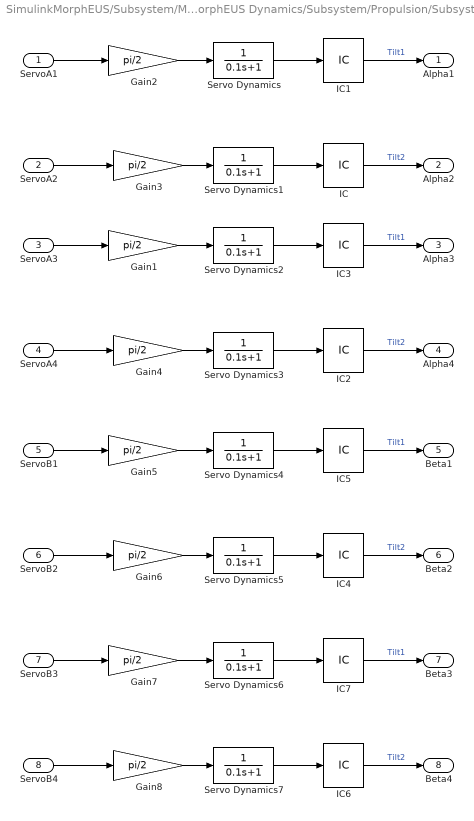
== system SimulinkMorphEUS/Subsystem/MorphEUS Dynamics/Subsystem/Propulsion/Subsystem ==
  ServoA1 : Inport
  ServoA2 : Inport  Port=2
  ServoA3 : Inport  Port=3
  ServoA4 : Inport  Port=4
  ServoB1 : Inport  Port=5
  ServoB2 : Inport  Port=6
  ServoB3 : Inport  Port=7
  ServoB4 : Inport  Port=8
  Gain{1..8} (8 alike) : Gain  Gain=pi/2
  IC{,1..7} (8 alike) : InitialCondition  Value=0
  Servo Dynamics{,1..7} (8 alike) : TransferFcn  Denominator=[0.1 1]
  Alpha1 : Outport
  Alpha2 : Outport  Port=2
  Alpha3 : Outport  Port=3
  Alpha4 : Outport  Port=4
  Beta1 : Outport  Port=5
  Beta2 : Outport  Port=6
  Beta3 : Outport  Port=7
  Beta4 : Outport  Port=8
  wires:
  ServoA1/1 -> Gain2/1
  Servo Dynamics1/1 -> IC/1
  Gain3/1 -> Servo Dynamics1/1
  Gain2/1 -> Servo Dynamics/1
  IC1/1 -> Alpha1/1  "Tilt1"
  Servo Dynamics/1 -> IC1/1
  IC/1 -> Alpha2/1  "Tilt2"
  ServoA2/1 -> Gain3/1
  IC2/1 -> Alpha4/1  "Tilt2"
  ServoA4/1 -> Gain4/1
  Gain1/1 -> Servo Dynamics2/1
  IC3/1 -> Alpha3/1  "Tilt1"
  Servo Dynamics2/1 -> IC3/1
  Servo Dynamics3/1 -> IC2/1
  Gain4/1 -> Servo Dynamics3/1
  ServoA3/1 -> Gain1/1
  IC4/1 -> Beta2/1  "Tilt2"
  ServoB2/1 -> Gain6/1
  Gain5/1 -> Servo Dynamics4/1
  IC5/1 -> Beta1/1  "Tilt1"
  Servo Dynamics4/1 -> IC5/1
  Servo Dynamics5/1 -> IC4/1
  Gain6/1 -> Servo Dynamics5/1
  ServoB1/1 -> Gain5/1
  IC6/1 -> Beta4/1  "Tilt2"
  ServoB4/1 -> Gain8/1
  Gain7/1 -> Servo Dynamics6/1
  IC7/1 -> Beta3/1  "Tilt1"
  Servo Dynamics6/1 -> IC7/1
  Servo Dynamics7/1 -> IC6/1
  Gain8/1 -> Servo Dynamics7/1
  ServoB3/1 -> Gain7/1

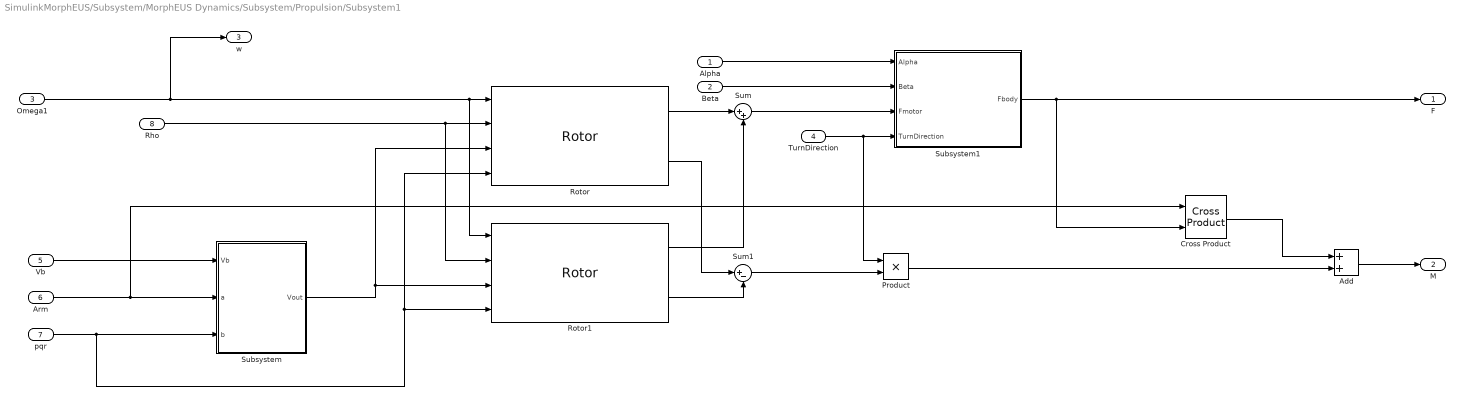
== system SimulinkMorphEUS/Subsystem/MorphEUS Dynamics/Subsystem/Propulsion/Subsystem1 ==
  Alpha : Inport
  "Beta " : Inport  Port=2
  Omega1 : Inport  Port=3
  TurnDirection : Inport  Port=4
  Vb : Inport  Port=5
  Arm : Inport  Port=6
  pqr : Inport  Port=7
  Rho : Inport  Port=8
  Add : Sum
  Cross Product : matrix_library/Cross Product
  Product : Product
  Rotor : Rotor  modelMode=With flap effects  CT=0.013  CQ=0.0013  Nb=3  radius=0.1016
  Rotor1 : Rotor  modelMode=With flap effects  CT=0.013  CQ=0.013  Nb=3  radius=0.1016
  Subsystem : Subsystem
  Subsystem1 : Subsystem
  Sum : Sum  Inputs=|++
  Sum1 : Sum  Inputs=|+-
  F : Outport
  M : Outport  Port=2
  w : Outport  Port=3
  wires:
  "Beta "/1 -> Subsystem1/2(Beta)
  Alpha/1 -> Subsystem1/1(Alpha)
  Add/1 -> M/1
  TurnDirection/1 -> Product/1, Subsystem1/4(TurnDirection)
  Cross Product/1 -> Add/1
  Rho/1 -> Rotor1/2, Rotor/2
  Rotor/1 -> Sum/1
  Rotor1/1 -> Sum/2
  Sum/1 -> Subsystem1/3(Fmotor)
  Rotor1/2 -> Sum1/2
  Sum1/1 -> Product/2
  Product/1 -> Add/2
  Subsystem1/1(Fbody) -> Cross Product/2, F/1
  Vb/1 -> Subsystem/1(Vb)
  pqr/1 -> Rotor1/4, Rotor/4, Subsystem/3(b)
  Subsystem/1(Vout) -> Rotor1/3, Rotor/3
  Arm/1 -> Cross Product/1, Subsystem/2(a)
  Omega1/1 -> Rotor1/1, Rotor/1, w/1
  Rotor/2 -> Sum1/1

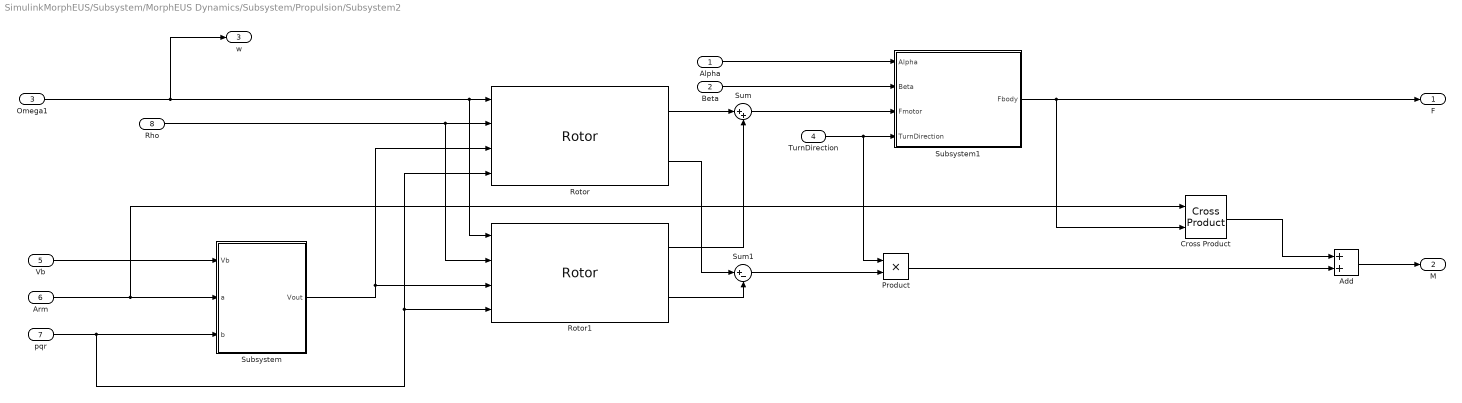
== system SimulinkMorphEUS/Subsystem/MorphEUS Dynamics/Subsystem/Propulsion/Subsystem2 ==
  Alpha : Inport
  "Beta " : Inport  Port=2
  Omega1 : Inport  Port=3
  TurnDirection : Inport  Port=4
  Vb : Inport  Port=5
  Arm : Inport  Port=6
  pqr : Inport  Port=7
  Rho : Inport  Port=8
  Add : Sum
  Cross Product : matrix_library/Cross Product
  Product : Product
  Rotor : Rotor  modelMode=With flap effects  CT=0.013  CQ=0.0013  Nb=3  radius=0.1016
  Rotor1 : Rotor  modelMode=With flap effects  CT=0.013  CQ=0.0013  Nb=3  radius=0.1016
  Subsystem : Subsystem
  Subsystem1 : Subsystem
  Sum : Sum  Inputs=|++
  Sum1 : Sum  Inputs=|+-
  F : Outport
  M : Outport  Port=2
  w : Outport  Port=3
  wires:
  "Beta "/1 -> Subsystem1/2(Beta)
  Alpha/1 -> Subsystem1/1(Alpha)
  Add/1 -> M/1
  TurnDirection/1 -> Product/1, Subsystem1/4(TurnDirection)
  Cross Product/1 -> Add/1
  Rho/1 -> Rotor1/2, Rotor/2
  Rotor/1 -> Sum/1
  Rotor1/1 -> Sum/2
  Sum/1 -> Subsystem1/3(Fmotor)
  Rotor1/2 -> Sum1/2
  Sum1/1 -> Product/2
  Product/1 -> Add/2
  Subsystem1/1(Fbody) -> Cross Product/2, F/1
  Vb/1 -> Subsystem/1(Vb)
  pqr/1 -> Rotor1/4, Rotor/4, Subsystem/3(b)
  Subsystem/1(Vout) -> Rotor1/3, Rotor/3
  Arm/1 -> Cross Product/1, Subsystem/2(a)
  Omega1/1 -> Rotor1/1, Rotor/1, w/1
  Rotor/2 -> Sum1/1

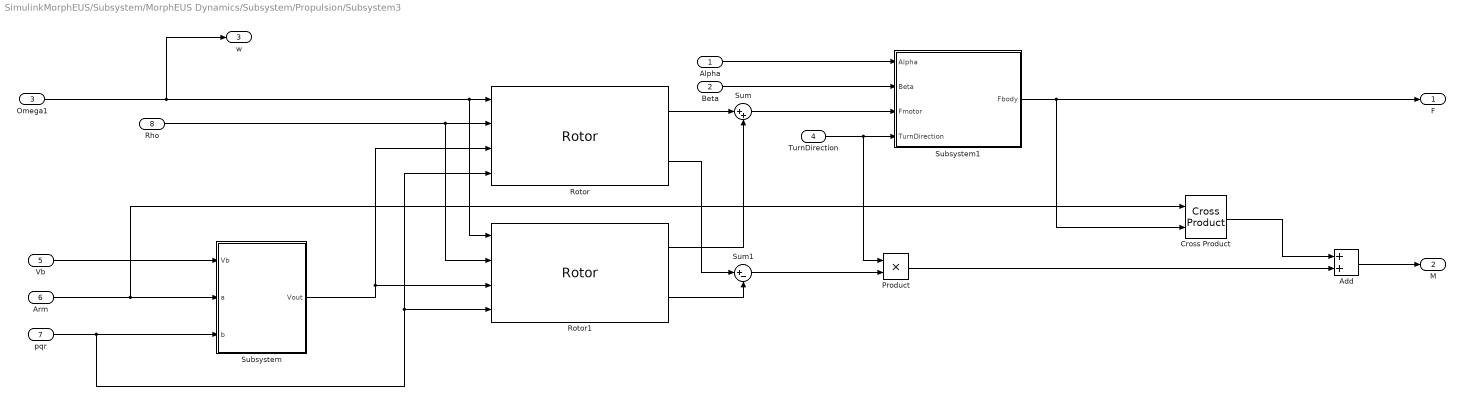
== system SimulinkMorphEUS/Subsystem/MorphEUS Dynamics/Subsystem/Propulsion/Subsystem3 ==
  Alpha : Inport
  "Beta " : Inport  Port=2
  Omega1 : Inport  Port=3
  TurnDirection : Inport  Port=4
  Vb : Inport  Port=5
  Arm : Inport  Port=6
  pqr : Inport  Port=7
  Rho : Inport  Port=8
  Add : Sum
  Cross Product : matrix_library/Cross Product
  Product : Product
  Rotor : Rotor  modelMode=With flap effects  CT=Ct  CQ=Cq  Nb=3  radius=0.1016
  Rotor1 : Rotor  modelMode=With flap effects  CT=Ct  CQ=Cq  Nb=3  radius=0.1016
  Subsystem : Subsystem
  Subsystem1 : Subsystem
  Sum : Sum  Inputs=|++
  Sum1 : Sum  Inputs=|+-
  F : Outport
  M : Outport  Port=2
  w : Outport  Port=3
  wires:
  "Beta "/1 -> Subsystem1/2(Beta)
  Alpha/1 -> Subsystem1/1(Alpha)
  Add/1 -> M/1
  TurnDirection/1 -> Product/1, Subsystem1/4(TurnDirection)
  Cross Product/1 -> Add/1
  Rho/1 -> Rotor1/2, Rotor/2
  Rotor/1 -> Sum/1
  Rotor1/1 -> Sum/2
  Sum/1 -> Subsystem1/3(Fmotor)
  Rotor1/2 -> Sum1/2
  Sum1/1 -> Product/2
  Product/1 -> Add/2
  Subsystem1/1(Fbody) -> Cross Product/2, F/1
  Vb/1 -> Subsystem/1(Vb)
  pqr/1 -> Rotor1/4, Rotor/4, Subsystem/3(b)
  Subsystem/1(Vout) -> Rotor1/3, Rotor/3
  Arm/1 -> Cross Product/1, Subsystem/2(a)
  Omega1/1 -> Rotor1/1, Rotor/1, w/1
  Rotor/2 -> Sum1/1

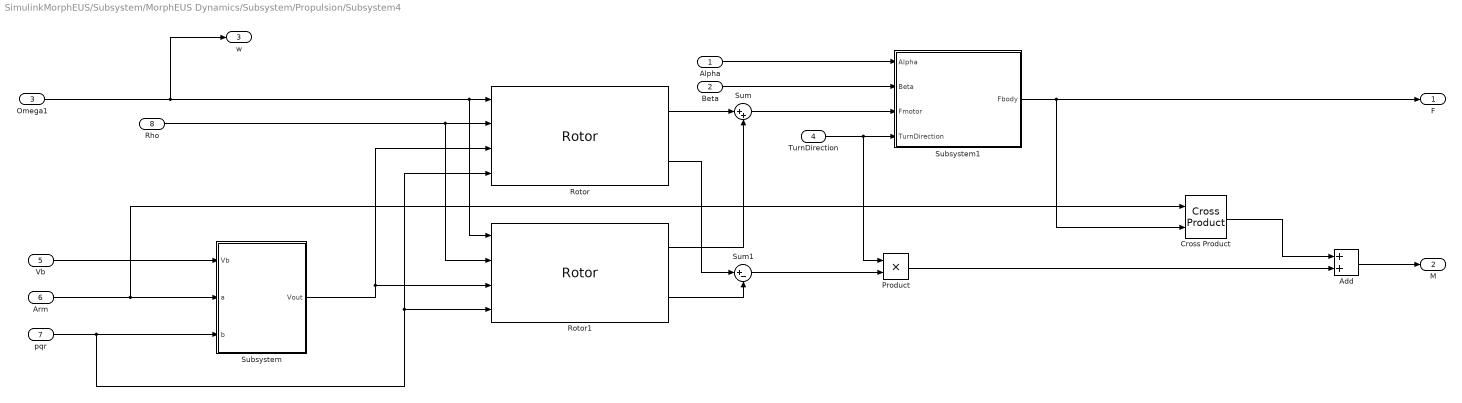
== system SimulinkMorphEUS/Subsystem/MorphEUS Dynamics/Subsystem/Propulsion/Subsystem4 ==
  Alpha : Inport
  "Beta " : Inport  Port=2
  Omega1 : Inport  Port=3
  TurnDirection : Inport  Port=4
  Vb : Inport  Port=5
  Arm : Inport  Port=6
  pqr : Inport  Port=7
  Rho : Inport  Port=8
  Add : Sum
  Cross Product : matrix_library/Cross Product
  Product : Product
  Rotor : Rotor  modelMode=With flap effects  CT=Ct  CQ=Cq  Nb=3  radius=0.1016
  Rotor1 : Rotor  modelMode=With flap effects  CT=Ct  CQ=Cq  Nb=3  radius=0.1016
  Subsystem : Subsystem
  Subsystem1 : Subsystem
  Sum : Sum  Inputs=|++
  Sum1 : Sum  Inputs=|+-
  F : Outport
  M : Outport  Port=2
  w : Outport  Port=3
  wires:
  "Beta "/1 -> Subsystem1/2(Beta)
  Alpha/1 -> Subsystem1/1(Alpha)
  Add/1 -> M/1
  TurnDirection/1 -> Product/1, Subsystem1/4(TurnDirection)
  Cross Product/1 -> Add/1
  Rho/1 -> Rotor1/2, Rotor/2
  Rotor/1 -> Sum/1
  Rotor1/1 -> Sum/2
  Sum/1 -> Subsystem1/3(Fmotor)
  Rotor1/2 -> Sum1/2
  Sum1/1 -> Product/2
  Product/1 -> Add/2
  Subsystem1/1(Fbody) -> Cross Product/2, F/1
  Vb/1 -> Subsystem/1(Vb)
  pqr/1 -> Rotor1/4, Rotor/4, Subsystem/3(b)
  Subsystem/1(Vout) -> Rotor1/3, Rotor/3
  Arm/1 -> Cross Product/1, Subsystem/2(a)
  Omega1/1 -> Rotor1/1, Rotor/1, w/1
  Rotor/2 -> Sum1/1

== system SimulinkMorphEUS/Subsystem/MorphEUS Dynamics/Subsystem/Ground Model/Friction Force/Soft Coulomb Friction ==
  note: Pennestrì, E., Rossi, V., Salvini, P. et al. Review and comparison of dry friction force models. Nonlinear Dyn 83, 1785–1801 (2016). https://doi.org/10.1007/s11071-015-2485-3
  V : Inport
  Tanh : Trigonometry  Operator=tanh
  friction coefficient : Gain  Gain=0.24
  vd : Gain  Gain=50
  Out1 : Outport
  wires:
  V/1 -> vd/1
  vd/1 -> Tanh/1
  Tanh/1 -> friction coefficient/1
  friction coefficient/1 -> Out1/1

== system SimulinkMorphEUS/Subsystem/MorphEUS Dynamics/Subsystem/Propulsion/Subsystem1/Subsystem ==
  Vb : Inport
  a : Inport  Port=2
  b : Inport  Port=3
  Cross Product : matrix_library/Cross Product
  Reshape : Reshape  OutputDimensionality=Column vector (2-D)
  Sum : Sum  Inputs=|++
  Vout : Outport
  wires:
  Vb/1 -> Reshape/1
  a/1 -> Cross Product/1
  b/1 -> Cross Product/2
  Reshape/1 -> Sum/1
  Cross Product/1 -> Sum/2
  Sum/1 -> Vout/1

== system SimulinkMorphEUS/Subsystem/MorphEUS Dynamics/Subsystem/Propulsion/Subsystem1/Subsystem1 ==
  Alpha : Inport
  Beta : Inport  Port=2
  Fmotor : Inport  Port=3
  TurnDirection : Inport  Port=4
  Constant : Constant  Value=0
  Constant1 : Constant
  Constant3 : Constant
  Coordinate Transformation Conversion : robotcorelib/Coordinate Transformation Conversion  InputRepresentation=Euler Angles  InputEulerSequence=ZYX  ShowTrVecInputPort=on  OutputRepresentation=Rotation Matrix  OutputEulerSequence=ZYX  ShowTrVecOutputPort=on  SimulateUsing=Interpreted execution
      settings: LibrarySourceBlock=uavutilslib/Coordinate Transformation Conversion
  MatrixMultiply : Product  Multiplication=Matrix(*)
  Mux : Mux  Inputs=3
  Mux1 : Mux  Inputs=3
  Product : Product
  Fbody : Outport
  wires:
  Constant/1 -> Mux/1
  Alpha/1 -> Mux/2
  Beta/1 -> Mux/3
  Mux/1 -> Coordinate Transformation Conversion/1
  Constant1/1 -> Mux1/1
  TurnDirection/1 -> Mux1/2
  Constant3/1 -> Mux1/3
  Fmotor/1 -> Product/1
  Mux1/1 -> Product/2
  Coordinate Transformation Conversion/1 -> MatrixMultiply/1
  Product/1 -> MatrixMultiply/2
  MatrixMultiply/1 -> Fbody/1

== system SimulinkMorphEUS/Subsystem/MorphEUS Dynamics/Subsystem/Propulsion/Subsystem2/Subsystem ==
  Vb : Inport
  a : Inport  Port=2
  b : Inport  Port=3
  Cross Product : matrix_library/Cross Product
  Reshape : Reshape  OutputDimensionality=Column vector (2-D)
  Sum : Sum  Inputs=|++
  Vout : Outport
  wires:
  Vb/1 -> Reshape/1
  a/1 -> Cross Product/1
  b/1 -> Cross Product/2
  Reshape/1 -> Sum/1
  Cross Product/1 -> Sum/2
  Sum/1 -> Vout/1

== system SimulinkMorphEUS/Subsystem/MorphEUS Dynamics/Subsystem/Propulsion/Subsystem2/Subsystem1 ==
  Alpha : Inport
  Beta : Inport  Port=2
  Fmotor : Inport  Port=3
  TurnDirection : Inport  Port=4
  Constant : Constant  Value=0
  Constant1 : Constant
  Constant3 : Constant
  Coordinate Transformation Conversion : robotcorelib/Coordinate Transformation Conversion  InputRepresentation=Euler Angles  InputEulerSequence=ZYX  ShowTrVecInputPort=on  OutputRepresentation=Rotation Matrix  OutputEulerSequence=ZYX  ShowTrVecOutputPort=on  SimulateUsing=Interpreted execution
      settings: LibrarySourceBlock=uavutilslib/Coordinate Transformation Conversion
  MatrixMultiply : Product  Multiplication=Matrix(*)
  Mux : Mux  Inputs=3
  Mux1 : Mux  Inputs=3
  Product : Product
  Fbody : Outport
  wires:
  Constant/1 -> Mux/1
  Alpha/1 -> Mux/2
  Beta/1 -> Mux/3
  Mux/1 -> Coordinate Transformation Conversion/1
  Constant1/1 -> Mux1/1
  TurnDirection/1 -> Mux1/2
  Constant3/1 -> Mux1/3
  Fmotor/1 -> Product/1
  Mux1/1 -> Product/2
  Coordinate Transformation Conversion/1 -> MatrixMultiply/1
  Product/1 -> MatrixMultiply/2
  MatrixMultiply/1 -> Fbody/1

== system SimulinkMorphEUS/Subsystem/MorphEUS Dynamics/Subsystem/Propulsion/Subsystem3/Subsystem ==
  Vb : Inport
  a : Inport  Port=2
  b : Inport  Port=3
  Cross Product : matrix_library/Cross Product
  Reshape : Reshape  OutputDimensionality=Column vector (2-D)
  Sum : Sum  Inputs=|++
  Vout : Outport
  wires:
  Vb/1 -> Reshape/1
  a/1 -> Cross Product/1
  b/1 -> Cross Product/2
  Reshape/1 -> Sum/1
  Cross Product/1 -> Sum/2
  Sum/1 -> Vout/1

== system SimulinkMorphEUS/Subsystem/MorphEUS Dynamics/Subsystem/Propulsion/Subsystem3/Subsystem1 ==
  Alpha : Inport
  Beta : Inport  Port=2
  Fmotor : Inport  Port=3
  TurnDirection : Inport  Port=4
  Constant : Constant  Value=0
  Constant1 : Constant
  Constant3 : Constant
  Coordinate Transformation Conversion : robotcorelib/Coordinate Transformation Conversion  InputRepresentation=Euler Angles  InputEulerSequence=ZYX  ShowTrVecInputPort=on  OutputRepresentation=Rotation Matrix  OutputEulerSequence=ZYX  ShowTrVecOutputPort=on  SimulateUsing=Interpreted execution
      settings: LibrarySourceBlock=uavutilslib/Coordinate Transformation Conversion
  MatrixMultiply : Product  Multiplication=Matrix(*)
  Mux : Mux  Inputs=3
  Mux1 : Mux  Inputs=3
  Product : Product
  Fbody : Outport
  wires:
  Constant/1 -> Mux/1
  Alpha/1 -> Mux/2
  Beta/1 -> Mux/3
  Mux/1 -> Coordinate Transformation Conversion/1
  Constant1/1 -> Mux1/1
  TurnDirection/1 -> Mux1/2
  Constant3/1 -> Mux1/3
  Fmotor/1 -> Product/1
  Mux1/1 -> Product/2
  Coordinate Transformation Conversion/1 -> MatrixMultiply/1
  Product/1 -> MatrixMultiply/2
  MatrixMultiply/1 -> Fbody/1

== system SimulinkMorphEUS/Subsystem/MorphEUS Dynamics/Subsystem/Propulsion/Subsystem4/Subsystem ==
  Vb : Inport
  a : Inport  Port=2
  b : Inport  Port=3
  Cross Product : matrix_library/Cross Product
  Reshape : Reshape  OutputDimensionality=Column vector (2-D)
  Sum : Sum  Inputs=|++
  Vout : Outport
  wires:
  Vb/1 -> Reshape/1
  a/1 -> Cross Product/1
  b/1 -> Cross Product/2
  Reshape/1 -> Sum/1
  Cross Product/1 -> Sum/2
  Sum/1 -> Vout/1

== system SimulinkMorphEUS/Subsystem/MorphEUS Dynamics/Subsystem/Propulsion/Subsystem4/Subsystem1 ==
  Alpha : Inport
  Beta : Inport  Port=2
  Fmotor : Inport  Port=3
  TurnDirection : Inport  Port=4
  Constant : Constant  Value=0
  Constant1 : Constant
  Constant3 : Constant
  Coordinate Transformation Conversion : robotcorelib/Coordinate Transformation Conversion  InputRepresentation=Euler Angles  InputEulerSequence=ZYX  ShowTrVecInputPort=on  OutputRepresentation=Rotation Matrix  OutputEulerSequence=ZYX  ShowTrVecOutputPort=on  SimulateUsing=Interpreted execution
      settings: LibrarySourceBlock=uavutilslib/Coordinate Transformation Conversion
  MatrixMultiply : Product  Multiplication=Matrix(*)
  Mux : Mux  Inputs=3
  Mux1 : Mux  Inputs=3
  Product : Product
  Fbody : Outport
  wires:
  Constant/1 -> Mux/1
  Alpha/1 -> Mux/2
  Beta/1 -> Mux/3
  Mux/1 -> Coordinate Transformation Conversion/1
  Constant1/1 -> Mux1/1
  TurnDirection/1 -> Mux1/2
  Constant3/1 -> Mux1/3
  Fmotor/1 -> Product/1
  Mux1/1 -> Product/2
  Coordinate Transformation Conversion/1 -> MatrixMultiply/1
  Product/1 -> MatrixMultiply/2
  MatrixMultiply/1 -> Fbody/1

== matlab function SimulinkMorphEUS/Subsystem3/MATLAB Function1 ==
  data: roll input; R_d output; pitch input; yaw input
function R_d = fcn(roll, pitch, yaw)

    Rx = [1, 0, 0;
          0, cos(roll), -sin(roll);
          0, sin(roll),  cos(roll)];
    Ry = [cos(pitch), 0, sin(pitch);
          0,       1,      0;
         -sin(pitch),0, cos(pitch)];
    Rz = [cos(yaw), -sin(yaw), 0;
          sin(yaw),  cos(yaw), 0;
          0,           0,    1];

    % Rd theo thứ tự Z * X * Y
    R_d = Rz * Rx * Ry;

== matlab function SimulinkMorphEUS/Subsystem/MorphEUS Dynamics/Feedback/MATLAB Function1 ==
  data: vxyz input; course output; gndSpeed output
function [course, gndSpeed] = fcn(vxyz)

vx = vxyz(1);
vy = vxyz(2);
course = atan2(vy, vx);
gndSpeed = norm([vx vy 0]);

== matlab function SimulinkMorphEUS/Subsystem/MorphEUS Dynamics/Subsystem/Aerodynamic Forces/Compute Air Data/MATLAB Function ==
  data: v input; F output
function F = fcn(v)
% Vb   : [3x1] vector vận tốc trong body frame (u,v,w) (m/s)
% rho  : mật độ không khí (kg/m^3)
% Cd   : hệ số cản (dimensionless)
% Af   : diện tích mặt cản tham chiếu (m^2)
% 
% F_drag : [3x1] vector lực cản trong body frame (N)
vx = v(1);
vy = v(2);
vz = v(3);

rho = 1.225;
Cd = 1;
Af = 0.04;
F = [0.5*rho*Cd*Af*vx^2 , 0.5*rho*Cd*Af*vy^2 , 0.5*rho*Cd*Af*vz^2];

== matlab function SimulinkMorphEUS/Subsystem/MorphEUS Dynamics/Ground Truth Bus/MATLAB Function1 ==
  data: vxyz input; course output; gndSpeed output
function [course, gndSpeed] = fcn(vxyz)

vx = vxyz(1);
vy = vxyz(2);
course = atan2(vy, vx);
gndSpeed = norm([vx vy 0]);

== matlab function SimulinkMorphEUS/Subsystem1/MATLAB Function ==
  data: R input; eR output; Rd input
function eR = RotationMatrixError(R, Rd)
% Compute attitude error vector eR between R and Rd
% Inputs:
%   R  - current rotation matrix (3x3)
%   Rd - desired rotation matrix (3x3)
% Output:
%   eR - attitude error vector (3x1)

% Skew-symmetric error matrix
E = 0.5 * (Rd' * R - R' * Rd);

% vee-map: extract vector from skew matrix
eR = [E(3,2); E(1,3); E(2,1)];
end

== matlab function SimulinkMorphEUS/Subsystem1/MATLAB Function1 ==
  data: R input; eOmega output; Rd input; omega input; omega_d input
function eOmega = omegaError(R, Rd, omega, omega_d)
% Compute angular velocity error eOmega
% Inputs:
%   R      - current rotation matrix (3x3)
%   Rd     - desired rotation matrix (3x3)
%   omega  - current angular velocity (3x1)
%   omega_d - desired angular velocity (3x1)
% Output:
%   eOmega - angular velocity error (3x1)

% Formula: e_omega = omega - R' * Rd * omega_d
eOmega = omega - R' * Rd * omega_d;
end

== matlab function SimulinkMorphEUS/Subsystem1/MATLAB Function2 ==
  data: R input; kpep input; fd output; kvev input; mg input; ma_d input; kReR input; kwew input; omega input; J input; R_d input; omega_d input; omega_d_dot input; tau_d output
function [fd, tau_d] = geometricController( R, kpep, ...
                                           kvev, mg, ma_d, kReR, kwew, omega, ...
                                           J, R_d, omega_d, omega_d_dot)
% Generalized Geometric Controller
% Inputs:
%   p, v      - current position (3x1), velocity (3x1)
%   R         - current rotation matrix (3x3)
%   omega     - current angular velocity (3x1)
%   pd, vd    - desired position, velocity (3x1)
%   ad        - desired acceleration (3x1)
%   Rd        - desired rotation matrix (3x3)
%   omegad    - desired angular velocity (3x1)
%   omegad_dot- desired angular acceleration (3x1)
%   m         - mass (scalar)
%   J         - inertia matrix (3x3)
%   kp, kv    - translational PD gains
%   kR, komega- rotational PD gains
%
% Outputs:
%   fd    - desired force (3x1, in body frame)
%   tau_d - desired torque (3x1, in body frame)
e3 = [0;0;1];
% --- Desired force ---
fd = -R' * (-kpep - kvev - mg*e3 + ma_d);
% --- Desired torque ---
tau_d = -kReR - kwew ...
        + cross(omega, J*omega) ...
        - J * ( cross(omega, R'*R_d*omega_d) ) ...
        - R' * R_d * omega_d_dot;
end
